simulink model "c28x_xcp_can_ext"  (R2021b)
settings: Solver=FixedStepDiscrete  StartTime=0.0  StopTime=Inf  RelTol=1e-3  EnableMultiTasking=on
libraries: demo_controls x1, simulink x1
settings Model: SimulationMode=external  ExtModeTrigDuration=8  Creator=The MathWorks, Inc.  LastModifiedBy=The MathWorks, Inc.
settings DataIOCC: ReturnWorkspaceOutputs=off
settings OptimizationCC: DefaultUnderspecifiedDataType=single  EnhancedBackFolding=on  PassReuseOutputArgsAs=Individual arguments  MaxStackSize=1024  OptimizeBlockOrder=speed  DifferentSizesBufferReuse=on  OptimizationCustomize=off  DenormalBehavior=FlushToZero  EfficientTunableParamExpr=on
settings DebuggingCC: ParameterPrecisionLossMsg=none  ParameterTunabilityLossMsg=error
settings HardwareCC: ProdBitPerChar=16  ProdBitPerInt=16  ProdBitPerPointer=32  ProdBitPerSizeT=32  ProdBitPerPtrDiffT=32  ProdLargestAtomicInteger=Integer  ProdLargestAtomicFloat=None  ProdWordSize=16  ProdLongLongMode=on  ProdHWDeviceType=Texas Instruments->C2000
settings ModelReferenceCC: ModelReferenceNumInstancesAllowed=Single
settings SFSimCC: MATLABDynamicMemAlloc=off
settings RTWCC: Description=Embedded Coder  SystemTargetFile=ert.tlc  HardwareBoard=TI F2838x (C28x)  TemplateMakefile=ert_default_tmf  Toolchain=Texas Instruments Code Composer Studio - EABI (C2000)
settings CodeAppCC: ForceParamTrailComments=on  IgnoreCustomStorageClasses=off  OperatorAnnotations=on  SimulinkDataObjDesc=on  SFDataObjDesc=on  InsertBlockDesc=on
settings ERTTargetCC: CodeReplacementLibrary=TI C28x  ExtModeTransport=5  ExtModeStaticAlloc=on  ExtModeStaticAllocSize=10000  ExtModeMexFile=ext_xcp  ExtModeIntrfLevel=Level2 - Open

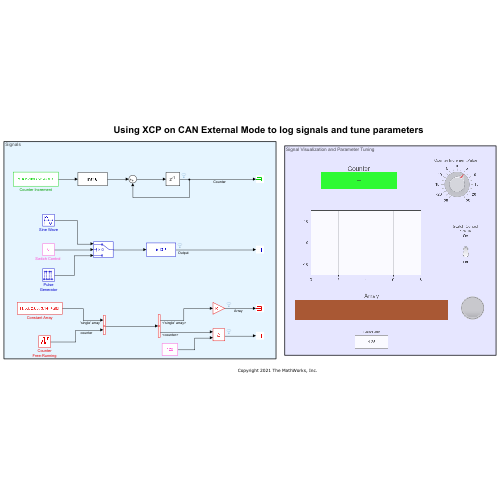
[thumbnail: Simulink's stored preview of the top-level diagram]
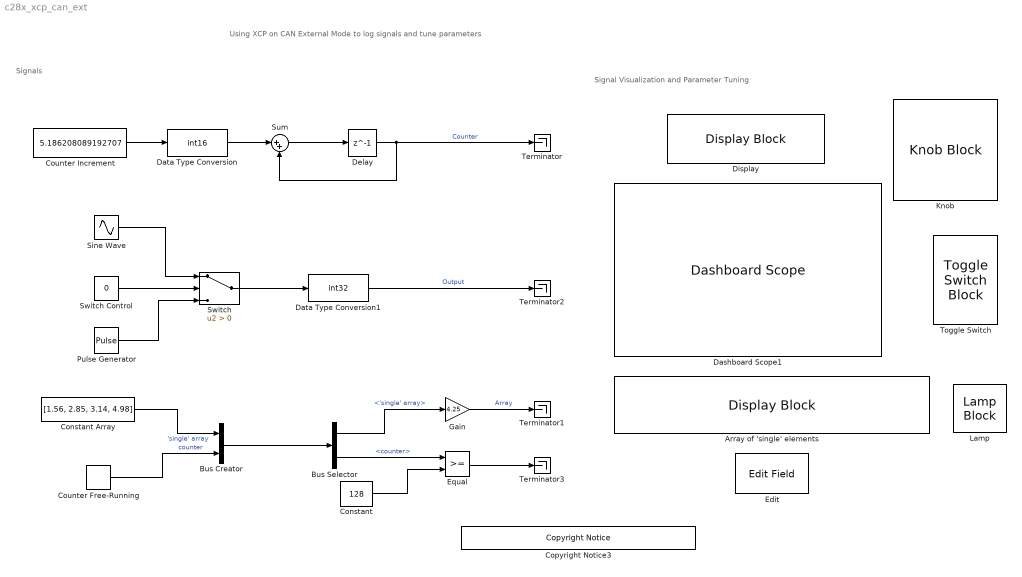
== system c28x_xcp_can_ext ==
  note: Signal Visualization and Parameter Tuning
  note: Signals
  note: Using XCP on CAN External Mode to log signals and tune parameters
  Array of 'single' elements : DisplayBlock  Format=short  Transparency=1  Layout=Fill available space
  Bus Creator : BusCreator  Inputs=2
  Bus Selector : BusSelector  OutputSignals='single' array,counter
  Constant : Constant  Value=128  OutDataTypeStr=uint8
  Constant Array : Constant  Value=[1.56, 2.85, 3.14, 4.98]  OutDataTypeStr=single  SampleTime=5e-3
  Copyright Notice3 : demo_controls/Copyright Notice  year=2021  prod=tic2000
      settings: SourceProductBaseCode=ME
  Counter Free-Running : simulink/Sources/Counter Free-Running  NumBits=8  tsamp=5e-3
  Counter Increment : Constant  Value=5.186208089192707  OutDataTypeStr=single  SampleTime=20e-3
  Dashboard Scope1 : DashboardScope  TimeSpan=8  Ymin=-15  Ymax=15
  Data Type Conversion : DataTypeConversion  OutDataTypeStr=int16
  Data Type Conversion1 : DataTypeConversion  OutDataTypeStr=int32
  Delay : Delay  DelayLength=1
  Display : DisplayBlock  Format=short  Transparency=1
  Edit : EditField  ShowInitialText=on  Alignment=Center
  Equal : RelationalOperator  OutDataTypeStr=boolean  RndMeth=Simplest
  Gain : Gain  Gain=4.25  OutDataTypeStr=single
  Knob : KnobBlock  ScaleMin=-25  ScaleMax=25
  Lamp : LampBlock  LabelPosition=Hide
  Pulse Generator : DiscretePulseGenerator  Amplitude=10  Period=30  PulseWidth=15  SampleTime=10e-3
  Sine Wave : Sin  SineType=Sample based  Amplitude=10  Samples=30  SampleTime=10e-3
  Sum : Sum  Inputs=|++
  Switch : Switch  Criteria=u2 > Threshold
  "Switch Control " : Constant  Value=0
  Terminator{,1..3} (4 alike) : Terminator
  Toggle Switch : ToggleSwitchBlock
      settings: Values={{'Off', 'On'}, [0 1]}
  wires:
  Pulse Generator/1 -> Switch/3
  "Switch Control "/1 -> Switch/2
  Switch/1 -> Data Type Conversion1/1
  Sine Wave/1 -> Switch/1
  Constant Array/1 -> Bus Creator/1  "'single' array"
  Counter Free-Running/1 -> Bus Creator/2  "counter"
  Data Type Conversion1/1 -> Terminator2/1  "Output"
  Bus Creator/1 -> Bus Selector/1
  Bus Selector/2 -> Equal/1  "<counter>"
  Constant/1 -> Equal/2
  Equal/1 -> Terminator3/1
  Bus Selector/1 -> Gain/1  "<'single' array>"
  Gain/1 -> Terminator1/1  "Array"
  Sum/1 -> Delay/1
  Delay/1 -> Terminator/1, Sum/2  "Counter"
  Counter Increment/1 -> Data Type Conversion/1
  Data Type Conversion/1 -> Sum/1
